simulink model "model"  (Simulink 8.7)
settings: Solver=FixedStepAuto  StartTime=0.0  StopTime=T  FixedStep=dt  RelTol=1e-3
values from neighbouring files (symbols this model uses):
  A = 0.05    [swarm.m]
  b = best_known_position(i, 2)    [swarm.m]
  f = 2*pi*15    (= 94.2477796077)    [swarm.m]
  g = 9.81    [swarm.m]
  k1 = best_known_position(i, 1)    [swarm.m]
  k2 = 200000    [swarm.m]
  m1 = 400    [swarm.m]
  m2 = 50    [swarm.m]
  u1 = -m1*g/k1+u2    (= -0.2182725)    [swarm.m]
  u2 = -(m1+m2)*g/k2    (= -0.0220725)    [swarm.m]
settings Model: Creator=Jakub  LastModifiedBy=Jakub
settings DataIOCC: LimitDataPoints=off  SaveFormat=Dataset
settings DebuggingCC: UnderspecifiedInitializationDetection=Simplified  MergeDetectMultiDrivingBlocksExec=error
settings HardwareCC: ProdBitPerPointer=64  ProdLargestAtomicFloat=Float  ProdIntDivRoundTo=Zero  ProdEndianess=LittleEndian  ProdWordSize=64  ProdHWDeviceType=Intel->x86-64 (Windows64)
settings ModelReferenceCC: PropagateSignalLabelsOutOfModel=on
settings ConfigComp: CovModelRefEnable=off

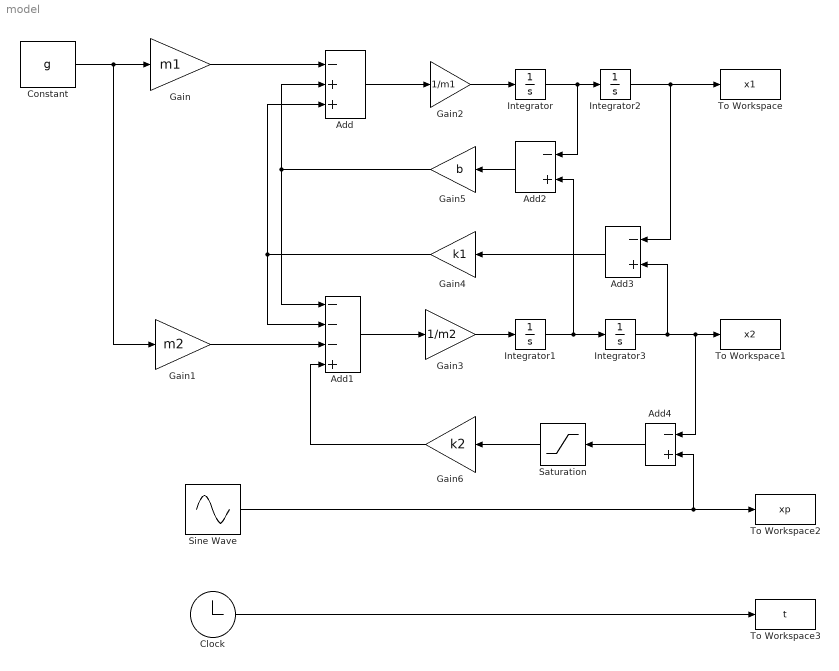
== system model ==
  Add : Sum  Inputs=-++
  Add1 : Sum  Inputs=---+
  Add2 : Sum  Inputs=-+
  Add3 : Sum  Inputs=-+
  Add4 : Sum  Inputs=-+
  Clock : Clock
  Constant : Constant  Value=g
  Gain : Gain  Gain=m1
  Gain1 : Gain  Gain=m2
  Gain2 : Gain  Gain=1/m1
  Gain3 : Gain  Gain=1/m2
  Gain4 : Gain  Gain=k1
  Gain5 : Gain  Gain=b
  Gain6 : Gain  Gain=k2
  Integrator : Integrator
  Integrator1 : Integrator
  Integrator2 : Integrator  InitialCondition=u1
  Integrator3 : Integrator  InitialCondition=u2
  Saturation : Saturate  UpperLimit=inf  LowerLimit=0
  Sine Wave : Sin  Amplitude=A  Frequency=f  SampleTime=0
  To Workspace : ToWorkspace  VariableName=x1  SampleTime=-1
  To Workspace1 : ToWorkspace  VariableName=x2  SampleTime=-1
  To Workspace2 : ToWorkspace  VariableName=xp  SampleTime=-1
  To Workspace3 : ToWorkspace  VariableName=t  SampleTime=-1
  wires:
  Gain2/1 -> Integrator/1
  Integrator/1 -> Add2/1, Integrator2/1
  Add1/1 -> Gain3/1
  Gain3/1 -> Integrator1/1
  Integrator1/1 -> Add2/2, Integrator3/1
  Integrator3/1 -> Add3/2, Add4/1, To Workspace1/1
  Integrator2/1 -> Add3/1, To Workspace/1
  Add/1 -> Gain2/1
  Add2/1 -> Gain5/1
  Add3/1 -> Gain4/1
  Gain5/1 -> Add1/1, Add/2
  Gain4/1 -> Add1/2, Add/3
  Gain/1 -> Add/1
  Gain1/1 -> Add1/3
  Gain6/1 -> Add1/4
  Saturation/1 -> Gain6/1
  Add4/1 -> Saturation/1
  Sine Wave/1 -> Add4/2, To Workspace2/1
  Clock/1 -> To Workspace3/1
  Constant/1 -> Gain1/1, Gain/1
